simulink model "KF_3_gdl_AHRS_Dataset2"  (R2020b)
settings: Solver=FixedStepAuto  StartTime=0.0  StopTime=1000  FixedStep=1/200  RelTol=1e-3
values from neighbouring files (symbols this model uses):
  BARO_cov = single(1.7)/2    [init_1gdl.m]    (also in init_3_gdl_AHRS_fb.m = single(1.7)/5; init_3gdl.m; init_dati_veri.m = single(1.7)/5)
  BARO_cov_old = single(1.7)/2    [init_1gdl.m]    (also in init_3_gdl_AHRS_fb.m; init_3gdl.m; init_dati_veri.m)
  bj_x = 0.4    [init_3_gdl_AHRS_fb.m]
  bj_y = 0.9    [init_3_gdl_AHRS_fb.m]
  bj_z = 0.5    [init_3_gdl_AHRS_fb.m]
  bjy = bj_y - 0.1    (= 0.8)    [init_3_gdl_AHRS_fb.m]
  filter_pos = tf(1,[1 1])    [init_1gdl.m]    (also in init_3_gdl_AHRS_fb.m; init_3gdl.m; init_dati_veri.m)
  filter_pos_Z = tf(1,[0.5 1])    [init_3_gdl_AHRS_fb.m]    (also in init_3gdl.m; init_dati_veri.m)
  g_ned = [0; 0; -9.81]    [init_3_gdl_AHRS_fb.m]    (also in init_dati_veri.m)
  GPS_cov = single([1*2, 1])/2    [init_1gdl.m]    (also in init_3_gdl_AHRS_fb.m = single([0.1*50, 0.1*50, 200*5, 200*5, 0.36])/2; init_3gdl.m = single([1*2, 1*2, 1, 1, 0.36])/2; init_dati_veri.m = single([0.1, 0.1, 200*5, 200*5, 0.36])/2)
  GPS_cov_old = single([0.1, 0.1, 200, 200, 0.36])/2    [init_1gdl.m]    (also in init_3_gdl_AHRS_fb.m = single([0.1, 0.1, 200, 200, 0.36]/2); init_3gdl.m; init_dati_veri.m = single([0.1, 0.1, 200, 200, 0.36]/2))
  IMU_cov = single(15*0.07)/2    [init_1gdl.m]    (also in init_3_gdl_AHRS_fb.m = single([15*[0.07*50, 0.07*50] 15*50*0.09])/2; init_3gdl.m = single([15*[0.07, 0.07] 10*0.09])/2; init_dati_veri.m = single([15*[0.07*5, 0.07*5] 15*50*0.09])/2)
  IMU_cov_old = single([15*[0.07, 0.07] 10*0.09])/2    [init_1gdl.m]    (also in init_3_gdl_AHRS_fb.m = single([15*[0.07, 0.07] 10*0.09]/2); init_3gdl.m; init_dati_veri.m = single([15*[0.07, 0.07] 10*0.09]/2))
  Q = single(diag([1e-2, 1e-6, 1e-4, 1e-12]))*2    [init_1gdl.m]    (also in init_3_gdl_AHRS_fb.m = single(diag([px,vx,ax,py,vy,ay,pz,vz,az,bx,by,bz]))*2; init_3gdl.m = single(diag([px,vx,ax,py,vy,ay,pz,vz,az,bx,by,bz]))*2; init_dati_veri.m = single(diag([px,vx,ax,py,vy,ay,pz,vz,az,bx,by,bz]))*2)
  Q_old = single(diag([1e-8, 1e-1, 1e-2, 1e-8, 1e-1, 1e-2, 1e-5, 1e-4, 0.010]))*2    [init_1gdl.m]    (also in init_3_gdl_AHRS_fb.m; init_3gdl.m; init_dati_veri.m)
  ST = 1/200    (= 0.005)    [init_1gdl.m]    (also in init_3_gdl_AHRS_fb.m; init_3gdl.m; init_dati_veri.m)
  T_50 = 1/50    (= 0.02)    [init_1gdl.m]    (also in init_3_gdl_AHRS_fb.m; init_3gdl.m; init_dati_veri.m)
  var_giroscopio = [(deg2rad(0.16))^2;(deg2rad(0.16))^2;(deg2rad(0.16))^2]    [init_3_gdl_AHRS_fb.m]    (also in init_dati_veri.m)
  var_p_x = 2    [init_3_gdl_AHRS_fb.m]    (also in init_3gdl.m = 1; init_dati_veri.m)
  var_p_y = 2    [init_3_gdl_AHRS_fb.m]    (also in init_3gdl.m = 1; init_dati_veri.m)
  var_p_z = 0.30    (= 0.3)    [init_3_gdl_AHRS_fb.m]    (also in init_3gdl.m = 0.15; init_dati_veri.m)
  var_v_x = 0.60    (= 0.6)    [init_3_gdl_AHRS_fb.m]    (also in init_3gdl.m = 0.3; init_dati_veri.m)
  var_v_y = 0.32    [init_3_gdl_AHRS_fb.m]    (also in init_3gdl.m = 0.16; init_dati_veri.m)
  var_v_z = 0.60    (= 0.6)    [init_3_gdl_AHRS_fb.m]    (also in init_3gdl.m = 0.3; init_dati_veri.m)
undefined symbols (not defined in the file or in its folder): DiscIntNeverNeededParam
libraries: simulink x33, cstblocks x9
(part 2 of 4)

== system KF_3_gdl_AHRS_Dataset2/MPU AHRS1/debias MPU ==
  acc : Inport
  gyros : Inport  Port=2
  "Acceleration Detrend " : Subsystem  mask{ST2=ST}
      mask prompts: ST2 "Sample Time"
  Add : Sum  Inputs=+-
  Data Type Conversion mx1 : DataTypeConversion  OutDataTypeStr=boolean  RndMeth=Round  SaturateOnIntegerOverflow=on
  Data Type Conversion mx8 : DataTypeConversion  OutDataTypeStr=single  RndMeth=Round  SaturateOnIntegerOverflow=on
  Gyros Detrend : Subsystem  mask{ST2=ST}
      mask prompts: ST2 "Sample Time"
  Step : Step  SampleTime=ST
  Step1 : Step  Time=11  SampleTime=ST
  acc_out : Outport
  gyro_out : Outport  Port=2
  detrending_ok : Outport  Port=3
  wires:
  Step/1 -> Add/1
  Step1/1 -> Add/2, Data Type Conversion mx1/1
  Add/1 -> Data Type Conversion mx8/1
  acc/1 -> "Acceleration Detrend "/1(In)
  gyros/1 -> Gyros Detrend/1(In)
  "Acceleration Detrend "/1(Out) -> acc_out/1
  Gyros Detrend/1(Out) -> gyro_out/1
  Data Type Conversion mx1/1 -> detrending_ok/1
  Data Type Conversion mx8/1 -> Gyros Detrend/2(Detrending), "Acceleration Detrend "/2(Detrending)

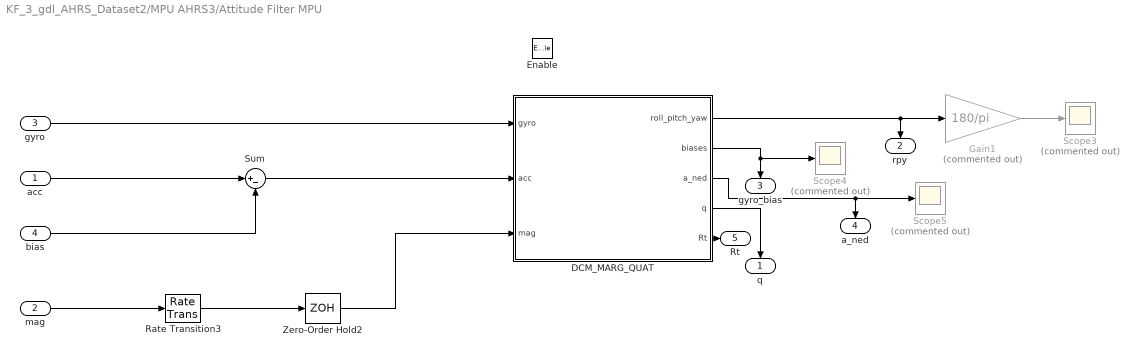
== system KF_3_gdl_AHRS_Dataset2/MPU AHRS3/Attitude Filter MPU ==
  acc : Inport
  mag : Inport  Port=2
  gyro : Inport  Port=3
  bias : Inport  Port=4
  Enable : EnablePort  StatesWhenEnabling=reset
  DCM_MARG_QUAT : Subsystem  mask{Kp=0.15*0, Ki=0, tau=40, T=T}
      mask prompts: Kp "Proportional Gain"; Ki "Integral Gain"; tau "Biases Time Constant"; T "Sample Time"
  Gain1 : Gain  Commented=on  Gain=180/pi
  Rate Transition3 : RateTransition  Deterministic=off
  Scope3 : Scope  Commented=on
  Scope4 : Scope  Commented=on
  Scope5 : Scope  Commented=on
  Sum : Sum  Inputs=|+-
  Zero-Order Hold2 : ZeroOrderHold  SampleTime=T
  q : Outport  PortDimensions=4  InitialOutput=[1 0 0 0]'
  rpy : Outport  Port=2  PortDimensions=3  InitialOutput=[0 0 0]'
  gyro_bias : Outport  Port=3  PortDimensions=3  InitialOutput=[0 0 0]'
  a_ned : Outport  Port=4  InitialOutput=[0 0 0]'
  Rt : Outport  Port=5
  wires:
  Rate Transition3/1 -> Zero-Order Hold2/1
  Zero-Order Hold2/1 -> DCM_MARG_QUAT/3(mag)
  DCM_MARG_QUAT/4(q) -> q/1
  bias/1 -> Sum/2
  Sum/1 -> DCM_MARG_QUAT/2(acc)
  acc/1 -> Sum/1
  DCM_MARG_QUAT/3(a_ned) -> a_ned/1, Scope5/1
  DCM_MARG_QUAT/1(roll_pitch_yaw) -> rpy/1, Gain1/1
  mag/1 -> Rate Transition3/1
  gyro/1 -> DCM_MARG_QUAT/1(gyro)
  DCM_MARG_QUAT/2(biases) -> gyro_bias/1, Scope4/1
  Gain1/1 -> Scope3/1
  DCM_MARG_QUAT/5(Rt) -> Rt/1

== system KF_3_gdl_AHRS_Dataset2/MPU AHRS3/debias MPU ==
  acc : Inport
  gyros : Inport  Port=2
  "Acceleration Detrend " : Subsystem  mask{ST2=ST}
      mask prompts: ST2 "Sample Time"
  Add : Sum  Inputs=+-
  Data Type Conversion mx1 : DataTypeConversion  OutDataTypeStr=boolean  RndMeth=Round  SaturateOnIntegerOverflow=on
  Data Type Conversion mx8 : DataTypeConversion  OutDataTypeStr=single  RndMeth=Round  SaturateOnIntegerOverflow=on
  Gyros Detrend : Subsystem  mask{ST2=ST}
      mask prompts: ST2 "Sample Time"
  Step : Step  SampleTime=ST
  Step1 : Step  Time=11  SampleTime=ST
  acc_out : Outport
  gyro_out : Outport  Port=2
  detrending_ok : Outport  Port=3
  wires:
  Step/1 -> Add/1
  Step1/1 -> Add/2, Data Type Conversion mx1/1
  Add/1 -> Data Type Conversion mx8/1
  acc/1 -> "Acceleration Detrend "/1(In)
  gyros/1 -> Gyros Detrend/1(In)
  "Acceleration Detrend "/1(Out) -> acc_out/1
  Gyros Detrend/1(Out) -> gyro_out/1
  Data Type Conversion mx8/1 -> "Acceleration Detrend "/2(Detrending), Gyros Detrend/2(Detrending)
  Data Type Conversion mx1/1 -> detrending_ok/1

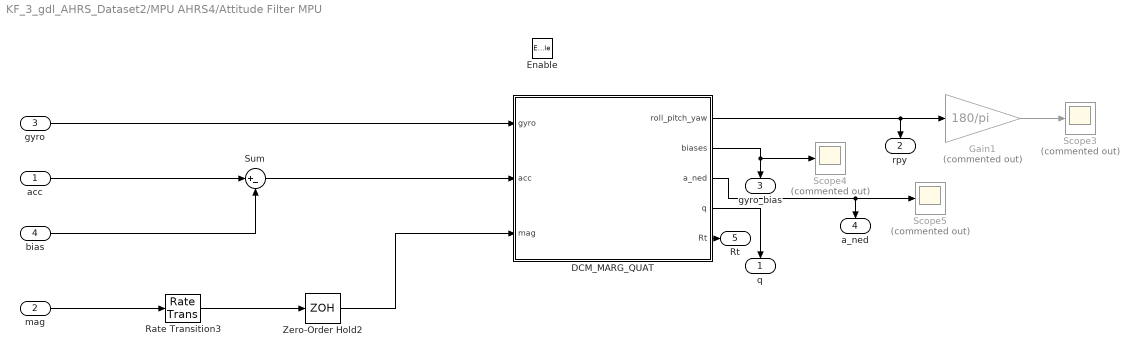
== system KF_3_gdl_AHRS_Dataset2/MPU AHRS4/Attitude Filter MPU ==
  acc : Inport
  mag : Inport  Port=2
  gyro : Inport  Port=3
  bias : Inport  Port=4
  Enable : EnablePort  StatesWhenEnabling=reset
  DCM_MARG_QUAT : Subsystem  mask{Kp=0.15, Ki=0, tau=40, T=T}
      mask prompts: Kp "Proportional Gain"; Ki "Integral Gain"; tau "Biases Time Constant"; T "Sample Time"
  Gain1 : Gain  Commented=on  Gain=180/pi
  Rate Transition3 : RateTransition  Deterministic=off
  Scope3 : Scope  Commented=on
  Scope4 : Scope  Commented=on
  Scope5 : Scope  Commented=on
  Sum : Sum  Inputs=|+-
  Zero-Order Hold2 : ZeroOrderHold  SampleTime=T
  q : Outport  PortDimensions=4  InitialOutput=[1 0 0 0]'
  rpy : Outport  Port=2  PortDimensions=3  InitialOutput=[0 0 0]'
  gyro_bias : Outport  Port=3  PortDimensions=3  InitialOutput=[0 0 0]'
  a_ned : Outport  Port=4  InitialOutput=[0 0 0]'
  Rt : Outport  Port=5
  wires:
  Rate Transition3/1 -> Zero-Order Hold2/1
  Zero-Order Hold2/1 -> DCM_MARG_QUAT/3(mag)
  DCM_MARG_QUAT/4(q) -> q/1
  bias/1 -> Sum/2
  Sum/1 -> DCM_MARG_QUAT/2(acc)
  acc/1 -> Sum/1
  DCM_MARG_QUAT/3(a_ned) -> a_ned/1, Scope5/1
  DCM_MARG_QUAT/1(roll_pitch_yaw) -> rpy/1, Gain1/1
  mag/1 -> Rate Transition3/1
  gyro/1 -> DCM_MARG_QUAT/1(gyro)
  DCM_MARG_QUAT/2(biases) -> gyro_bias/1, Scope4/1
  Gain1/1 -> Scope3/1
  DCM_MARG_QUAT/5(Rt) -> Rt/1

== system KF_3_gdl_AHRS_Dataset2/MPU AHRS4/debias MPU ==
  acc : Inport
  gyros : Inport  Port=2
  "Acceleration Detrend " : Subsystem  mask{ST2=ST}
      mask prompts: ST2 "Sample Time"
  Add : Sum  Inputs=+-
  Data Type Conversion mx1 : DataTypeConversion  OutDataTypeStr=boolean  RndMeth=Round  SaturateOnIntegerOverflow=on
  Data Type Conversion mx8 : DataTypeConversion  OutDataTypeStr=single  RndMeth=Round  SaturateOnIntegerOverflow=on
  Gyros Detrend : Subsystem  mask{ST2=ST}
      mask prompts: ST2 "Sample Time"
  Step : Step  SampleTime=ST
  Step1 : Step  Time=11  SampleTime=ST
  acc_out : Outport
  gyro_out : Outport  Port=2
  detrending_ok : Outport  Port=3
  wires:
  Step/1 -> Add/1
  Step1/1 -> Add/2, Data Type Conversion mx1/1
  Add/1 -> Data Type Conversion mx8/1
  acc/1 -> "Acceleration Detrend "/1(In)
  gyros/1 -> Gyros Detrend/1(In)
  "Acceleration Detrend "/1(Out) -> acc_out/1
  Gyros Detrend/1(Out) -> gyro_out/1
  Data Type Conversion mx1/1 -> detrending_ok/1
  Data Type Conversion mx8/1 -> Gyros Detrend/2(Detrending), "Acceleration Detrend "/2(Detrending)

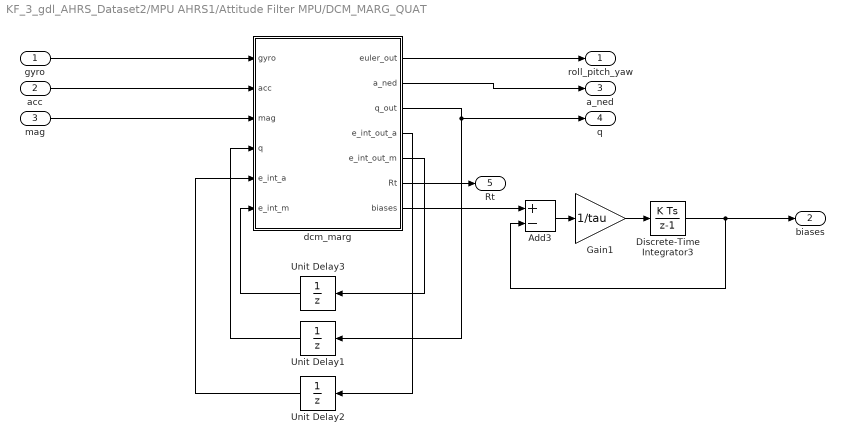
== system KF_3_gdl_AHRS_Dataset2/MPU AHRS1/Attitude Filter MPU/DCM_MARG_QUAT ==
  gyro : Inport
  acc : Inport  Port=2
  mag : Inport  Port=3
  Add3 : Sum  Inputs=+-
  Discrete-Time Integrator3 : DiscreteIntegrator  SampleTime=T  ICPrevOutput=DiscIntNeverNeededParam  ICPrevScaledInput=DiscIntNeverNeededParam
  Gain1 : Gain  Gain=1/tau  ParamDataTypeStr=single  OutDataTypeStr=single
  Unit Delay1 : UnitDelay  InitialCondition=[1;0;0;0]  SampleTime=T  HasFrameUpgradeWarning=on
  Unit Delay2 : UnitDelay  SampleTime=T  HasFrameUpgradeWarning=on
  Unit Delay3 : UnitDelay  SampleTime=T  HasFrameUpgradeWarning=on
  dcm_marg : MATLAB Function  TreatAsAtomicUnit=on
  roll_pitch_yaw : Outport
  biases : Outport  Port=2
  a_ned : Outport  Port=3
  q : Outport  Port=4
  Rt : Outport  Port=5
  wires:
  Unit Delay3/1 -> dcm_marg/6(e_int_m)
  dcm_marg/5(e_int_out_m) -> Unit Delay3/1
  dcm_marg/2(a_ned) -> a_ned/1
  Discrete-Time Integrator3/1 -> biases/1, Add3/2
  Gain1/1 -> Discrete-Time Integrator3/1
  Add3/1 -> Gain1/1
  dcm_marg/1(euler_out) -> roll_pitch_yaw/1
  gyro/1 -> dcm_marg/1(gyro)
  acc/1 -> dcm_marg/2(acc)
  mag/1 -> dcm_marg/3(mag)
  dcm_marg/3(q_out) -> q/1, Unit Delay1/1
  Unit Delay1/1 -> dcm_marg/4(q)
  dcm_marg/4(e_int_out_a) -> Unit Delay2/1
  Unit Delay2/1 -> dcm_marg/5(e_int_a)
  dcm_marg/7(biases) -> Add3/1
  dcm_marg/6(Rt) -> Rt/1

== system KF_3_gdl_AHRS_Dataset2/MPU AHRS1/debias MPU/Acceleration Detrend  ==
  In : Inport
  Detrending : Inport  Port=2
  Demux : Demux  Outputs=3
      settings: DisplayOption=none
  Detrend : Subsystem  mask{ST=ST2}
      mask prompts: ST "Sample Time"
  Detrend1 : Subsystem  mask{ST=ST2}
      mask prompts: ST "Sample Time"
  Detrend3 : Subsystem  mask{ST=ST2}
      mask prompts: ST "Sample Time"
  Mux : Mux  Inputs=3
  Out : Outport
  wires:
  Detrending/1 -> Detrend3/2(Detrending), Detrend1/2(Detrending), Detrend/2(Detrending)
  Demux/3 -> Detrend3/1(Input)
  In/1 -> Demux/1
  Demux/2 -> Detrend1/1(Input)
  Demux/1 -> Detrend/1(Input)
  Mux/1 -> Out/1
  Detrend3/1(Detrended Output) -> Mux/3
  Detrend1/1(Detrended Output) -> Mux/2
  Detrend/1(Detrended Output) -> Mux/1

== system KF_3_gdl_AHRS_Dataset2/MPU AHRS1/debias MPU/Gyros Detrend ==
  In : Inport
  Detrending : Inport  Port=2
  Demux : Demux  Outputs=3
      settings: DisplayOption=none
  Detrend : Subsystem  mask{ST=ST2}
      mask prompts: ST "Sample Time"
  Detrend2 : Subsystem  mask{ST=ST2}
      mask prompts: ST "Sample Time"
  Detrend3 : Subsystem  mask{ST=ST2}
      mask prompts: ST "Sample Time"
  Mux : Mux  Inputs=3
  Out : Outport
  wires:
  Detrend/1(Detrended Output) -> Mux/1
  Detrend3/1(Detrended Output) -> Mux/2
  Detrend2/1(Detrended Output) -> Mux/3
  Mux/1 -> Out/1
  Demux/1 -> Detrend/1(Input)
  Demux/2 -> Detrend3/1(Input)
  In/1 -> Demux/1
  Demux/3 -> Detrend2/1(Input)
  Detrending/1 -> Detrend2/2(Detrending), Detrend3/2(Detrending), Detrend/2(Detrending)

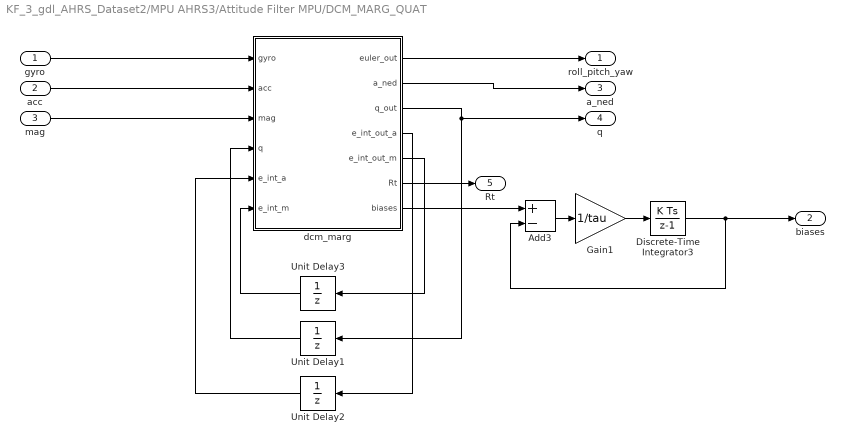
== system KF_3_gdl_AHRS_Dataset2/MPU AHRS3/Attitude Filter MPU/DCM_MARG_QUAT ==
  gyro : Inport
  acc : Inport  Port=2
  mag : Inport  Port=3
  Add3 : Sum  Inputs=+-
  Discrete-Time Integrator3 : DiscreteIntegrator  SampleTime=T  ICPrevOutput=DiscIntNeverNeededParam  ICPrevScaledInput=DiscIntNeverNeededParam
  Gain1 : Gain  Gain=1/tau  ParamDataTypeStr=single  OutDataTypeStr=single
  Unit Delay1 : UnitDelay  InitialCondition=[1;0;0;0]  SampleTime=T  HasFrameUpgradeWarning=on
  Unit Delay2 : UnitDelay  SampleTime=T  HasFrameUpgradeWarning=on
  Unit Delay3 : UnitDelay  SampleTime=T  HasFrameUpgradeWarning=on
  dcm_marg : MATLAB Function  TreatAsAtomicUnit=on
  roll_pitch_yaw : Outport
  biases : Outport  Port=2
  a_ned : Outport  Port=3
  q : Outport  Port=4
  Rt : Outport  Port=5
  wires:
  Unit Delay3/1 -> dcm_marg/6(e_int_m)
  dcm_marg/5(e_int_out_m) -> Unit Delay3/1
  dcm_marg/2(a_ned) -> a_ned/1
  Discrete-Time Integrator3/1 -> biases/1, Add3/2
  Gain1/1 -> Discrete-Time Integrator3/1
  Add3/1 -> Gain1/1
  dcm_marg/1(euler_out) -> roll_pitch_yaw/1
  gyro/1 -> dcm_marg/1(gyro)
  acc/1 -> dcm_marg/2(acc)
  mag/1 -> dcm_marg/3(mag)
  dcm_marg/3(q_out) -> q/1, Unit Delay1/1
  Unit Delay1/1 -> dcm_marg/4(q)
  dcm_marg/4(e_int_out_a) -> Unit Delay2/1
  Unit Delay2/1 -> dcm_marg/5(e_int_a)
  dcm_marg/7(biases) -> Add3/1
  dcm_marg/6(Rt) -> Rt/1

== system KF_3_gdl_AHRS_Dataset2/MPU AHRS3/debias MPU/Acceleration Detrend  ==
  In : Inport
  Detrending : Inport  Port=2
  Demux : Demux  Outputs=3
      settings: DisplayOption=none
  Detrend : Subsystem  mask{ST=ST2}
      mask prompts: ST "Sample Time"
  Detrend1 : Subsystem  mask{ST=ST2}
      mask prompts: ST "Sample Time"
  Detrend3 : Subsystem  mask{ST=ST2}
      mask prompts: ST "Sample Time"
  Mux : Mux  Inputs=3
  Out : Outport
  wires:
  Detrending/1 -> Detrend3/2(Detrending), Detrend1/2(Detrending), Detrend/2(Detrending)
  Demux/3 -> Detrend3/1(Input)
  In/1 -> Demux/1
  Demux/2 -> Detrend1/1(Input)
  Demux/1 -> Detrend/1(Input)
  Mux/1 -> Out/1
  Detrend3/1(Detrended Output) -> Mux/3
  Detrend1/1(Detrended Output) -> Mux/2
  Detrend/1(Detrended Output) -> Mux/1

== system KF_3_gdl_AHRS_Dataset2/MPU AHRS3/debias MPU/Gyros Detrend ==
  In : Inport
  Detrending : Inport  Port=2
  Demux : Demux  Outputs=3
      settings: DisplayOption=none
  Detrend : Subsystem  mask{ST=ST2}
      mask prompts: ST "Sample Time"
  Detrend2 : Subsystem  mask{ST=ST2}
      mask prompts: ST "Sample Time"
  Detrend3 : Subsystem  mask{ST=ST2}
      mask prompts: ST "Sample Time"
  Mux : Mux  Inputs=3
  Out : Outport
  wires:
  Detrend/1(Detrended Output) -> Mux/1
  Detrend3/1(Detrended Output) -> Mux/2
  Detrend2/1(Detrended Output) -> Mux/3
  Mux/1 -> Out/1
  Demux/1 -> Detrend/1(Input)
  Demux/2 -> Detrend3/1(Input)
  In/1 -> Demux/1
  Demux/3 -> Detrend2/1(Input)
  Detrending/1 -> Detrend2/2(Detrending), Detrend3/2(Detrending), Detrend/2(Detrending)

== system KF_3_gdl_AHRS_Dataset2/MPU AHRS4/Attitude Filter MPU/DCM_MARG_QUAT ==
  gyro : Inport
  acc : Inport  Port=2
  mag : Inport  Port=3
  Add3 : Sum  Inputs=+-
  Discrete-Time Integrator3 : DiscreteIntegrator  SampleTime=T  ICPrevOutput=DiscIntNeverNeededParam  ICPrevScaledInput=DiscIntNeverNeededParam
  Gain1 : Gain  Gain=1/tau  ParamDataTypeStr=single  OutDataTypeStr=single
  Unit Delay1 : UnitDelay  InitialCondition=[1;0;0;0]  SampleTime=T  HasFrameUpgradeWarning=on
  Unit Delay2 : UnitDelay  SampleTime=T  HasFrameUpgradeWarning=on
  Unit Delay3 : UnitDelay  SampleTime=T  HasFrameUpgradeWarning=on
  dcm_marg : MATLAB Function  TreatAsAtomicUnit=on
  roll_pitch_yaw : Outport
  biases : Outport  Port=2
  a_ned : Outport  Port=3
  q : Outport  Port=4
  Rt : Outport  Port=5
  wires:
  Unit Delay3/1 -> dcm_marg/6(e_int_m)
  dcm_marg/5(e_int_out_m) -> Unit Delay3/1
  dcm_marg/2(a_ned) -> a_ned/1
  Discrete-Time Integrator3/1 -> biases/1, Add3/2
  Gain1/1 -> Discrete-Time Integrator3/1
  Add3/1 -> Gain1/1
  dcm_marg/1(euler_out) -> roll_pitch_yaw/1
  gyro/1 -> dcm_marg/1(gyro)
  acc/1 -> dcm_marg/2(acc)
  mag/1 -> dcm_marg/3(mag)
  dcm_marg/3(q_out) -> q/1, Unit Delay1/1
  Unit Delay1/1 -> dcm_marg/4(q)
  dcm_marg/4(e_int_out_a) -> Unit Delay2/1
  Unit Delay2/1 -> dcm_marg/5(e_int_a)
  dcm_marg/7(biases) -> Add3/1
  dcm_marg/6(Rt) -> Rt/1

== system KF_3_gdl_AHRS_Dataset2/MPU AHRS4/debias MPU/Acceleration Detrend  ==
  In : Inport
  Detrending : Inport  Port=2
  Demux : Demux  Outputs=3
      settings: DisplayOption=none
  Detrend : Subsystem  mask{ST=ST2}
      mask prompts: ST "Sample Time"
  Detrend1 : Subsystem  mask{ST=ST2}
      mask prompts: ST "Sample Time"
  Detrend3 : Subsystem  mask{ST=ST2}
      mask prompts: ST "Sample Time"
  Mux : Mux  Inputs=3
  Out : Outport
  wires:
  Detrending/1 -> Detrend3/2(Detrending), Detrend1/2(Detrending), Detrend/2(Detrending)
  Demux/3 -> Detrend3/1(Input)
  In/1 -> Demux/1
  Demux/2 -> Detrend1/1(Input)
  Demux/1 -> Detrend/1(Input)
  Mux/1 -> Out/1
  Detrend3/1(Detrended Output) -> Mux/3
  Detrend1/1(Detrended Output) -> Mux/2
  Detrend/1(Detrended Output) -> Mux/1

== system KF_3_gdl_AHRS_Dataset2/MPU AHRS4/debias MPU/Gyros Detrend ==
  In : Inport
  Detrending : Inport  Port=2
  Demux : Demux  Outputs=3
      settings: DisplayOption=none
  Detrend : Subsystem  mask{ST=ST2}
      mask prompts: ST "Sample Time"
  Detrend2 : Subsystem  mask{ST=ST2}
      mask prompts: ST "Sample Time"
  Detrend3 : Subsystem  mask{ST=ST2}
      mask prompts: ST "Sample Time"
  Mux : Mux  Inputs=3
  Out : Outport
  wires:
  Detrend/1(Detrended Output) -> Mux/1
  Detrend3/1(Detrended Output) -> Mux/2
  Detrend2/1(Detrended Output) -> Mux/3
  Mux/1 -> Out/1
  Demux/1 -> Detrend/1(Input)
  Demux/2 -> Detrend3/1(Input)
  In/1 -> Demux/1
  Demux/3 -> Detrend2/1(Input)
  Detrending/1 -> Detrend2/2(Detrending), Detrend3/2(Detrending), Detrend/2(Detrending)

== system KF_3_gdl_AHRS_Dataset2/MPU AHRS1/debias MPU/Acceleration Detrend /Detrend ==
  Input : Inport
  Detrending : Inport  Port=2
  Compare To Constant : simulink/Logic and Bit Operations/Compare To Constant  relop=>=  const=0.5  OutDataTypeStr=boolean
  Constant1 : Constant  Value=0  OutDataTypeStr=single
  Subsystem : Subsystem  TreatAsAtomicUnit=on
  Sum1 : Sum  Inputs=|+-  InputSameDT=on  SaturateOnIntegerOverflow=on  OutDataTypeStr=Inherit: Same as first input
  Switch2 : Switch  Threshold=0.5  SaturateOnIntegerOverflow=on  InputSameDT=on
  Detrended Output : Outport
  wires:
  Switch2/1 -> Detrended Output/1
  Detrending/1 -> Switch2/2, Compare To Constant/1
  Subsystem/1(Out2) -> Sum1/2
  Constant1/1 -> Switch2/1
  Input/1 -> Sum1/1, Subsystem/1(In1)
  Sum1/1 -> Switch2/3
  Compare To Constant/1 -> Subsystem/Enable

== system KF_3_gdl_AHRS_Dataset2/MPU AHRS1/debias MPU/Acceleration Detrend /Detrend1 ==
  Input : Inport
  Detrending : Inport  Port=2
  Compare To Constant : simulink/Logic and Bit Operations/Compare To Constant  relop=>=  const=0.5  OutDataTypeStr=boolean
  Constant1 : Constant  Value=0  OutDataTypeStr=single
  Subsystem : Subsystem  TreatAsAtomicUnit=on
  Sum1 : Sum  Inputs=|+-  InputSameDT=on  SaturateOnIntegerOverflow=on  OutDataTypeStr=Inherit: Same as first input
  Switch2 : Switch  Threshold=0.5  SaturateOnIntegerOverflow=on  InputSameDT=on
  Detrended Output : Outport
  wires:
  Compare To Constant/1 -> Subsystem/Enable
  Sum1/1 -> Switch2/3
  Input/1 -> Subsystem/1(In1), Sum1/1
  Constant1/1 -> Switch2/1
  Subsystem/1(Out2) -> Sum1/2
  Detrending/1 -> Compare To Constant/1, Switch2/2
  Switch2/1 -> Detrended Output/1

== system KF_3_gdl_AHRS_Dataset2/MPU AHRS1/debias MPU/Acceleration Detrend /Detrend3 ==
  Input : Inport
  Detrending : Inport  Port=2
  Compare To Constant : simulink/Logic and Bit Operations/Compare To Constant  relop=>=  const=0.5  OutDataTypeStr=boolean
  Constant1 : Constant  Value=0  OutDataTypeStr=single
  Constant2 : Constant  Value=9.81  OutDataTypeStr=single
  Subsystem : Subsystem  TreatAsAtomicUnit=on
  Sum1 : Sum  Inputs=|+--  InputSameDT=on  SaturateOnIntegerOverflow=on  OutDataTypeStr=Inherit: Same as first input
  Switch2 : Switch  Threshold=0.5  SaturateOnIntegerOverflow=on  InputSameDT=on
  Detrended Output : Outport
  wires:
  Switch2/1 -> Detrended Output/1
  Detrending/1 -> Switch2/2, Compare To Constant/1
  Subsystem/1(Out2) -> Sum1/2
  Constant1/1 -> Switch2/1
  Input/1 -> Sum1/1, Subsystem/1(In1)
  Sum1/1 -> Switch2/3
  Compare To Constant/1 -> Subsystem/Enable
  Constant2/1 -> Sum1/3

== system KF_3_gdl_AHRS_Dataset2/MPU AHRS1/debias MPU/Gyros Detrend/Detrend ==
  Input : Inport
  Detrending : Inport  Port=2
  Compare To Constant : simulink/Logic and Bit Operations/Compare To Constant  relop=>=  const=0.5  OutDataTypeStr=boolean
  Constant1 : Constant  Value=0  OutDataTypeStr=single
  Subsystem : Subsystem  TreatAsAtomicUnit=on
  Sum1 : Sum  Inputs=|+-  InputSameDT=on  SaturateOnIntegerOverflow=on  OutDataTypeStr=Inherit: Same as first input
  Switch2 : Switch  Threshold=0.5  SaturateOnIntegerOverflow=on  InputSameDT=on
  Detrended Output : Outport
  wires:
  Switch2/1 -> Detrended Output/1
  Detrending/1 -> Switch2/2, Compare To Constant/1
  Subsystem/1(Out2) -> Sum1/2
  Constant1/1 -> Switch2/1
  Input/1 -> Sum1/1, Subsystem/1(In1)
  Sum1/1 -> Switch2/3
  Compare To Constant/1 -> Subsystem/Enable

== system KF_3_gdl_AHRS_Dataset2/MPU AHRS1/debias MPU/Gyros Detrend/Detrend2 ==
  Input : Inport
  Detrending : Inport  Port=2
  Compare To Constant : simulink/Logic and Bit Operations/Compare To Constant  relop=>=  const=0.5  OutDataTypeStr=boolean
  Constant1 : Constant  Value=0  OutDataTypeStr=single
  Subsystem : Subsystem  TreatAsAtomicUnit=on
  Sum1 : Sum  Inputs=|+-  InputSameDT=on  SaturateOnIntegerOverflow=on  OutDataTypeStr=Inherit: Same as first input
  Switch2 : Switch  Threshold=0.5  SaturateOnIntegerOverflow=on  InputSameDT=on
  Detrended Output : Outport
  wires:
  Switch2/1 -> Detrended Output/1
  Detrending/1 -> Switch2/2, Compare To Constant/1
  Subsystem/1(Out2) -> Sum1/2
  Constant1/1 -> Switch2/1
  Input/1 -> Sum1/1, Subsystem/1(In1)
  Sum1/1 -> Switch2/3
  Compare To Constant/1 -> Subsystem/Enable

== system KF_3_gdl_AHRS_Dataset2/MPU AHRS1/debias MPU/Gyros Detrend/Detrend3 ==
  Input : Inport
  Detrending : Inport  Port=2
  Compare To Constant : simulink/Logic and Bit Operations/Compare To Constant  relop=>=  const=0.5  OutDataTypeStr=boolean
  Constant1 : Constant  Value=0  OutDataTypeStr=single
  Subsystem : Subsystem  TreatAsAtomicUnit=on
  Sum1 : Sum  Inputs=|+-  InputSameDT=on  SaturateOnIntegerOverflow=on  OutDataTypeStr=Inherit: Same as first input
  Switch2 : Switch  Threshold=0.5  SaturateOnIntegerOverflow=on  InputSameDT=on
  Detrended Output : Outport
  wires:
  Compare To Constant/1 -> Subsystem/Enable
  Sum1/1 -> Switch2/3
  Input/1 -> Subsystem/1(In1), Sum1/1
  Constant1/1 -> Switch2/1
  Subsystem/1(Out2) -> Sum1/2
  Detrending/1 -> Compare To Constant/1, Switch2/2
  Switch2/1 -> Detrended Output/1

== system KF_3_gdl_AHRS_Dataset2/MPU AHRS3/debias MPU/Acceleration Detrend /Detrend ==
  Input : Inport
  Detrending : Inport  Port=2
  Compare To Constant : simulink/Logic and Bit Operations/Compare To Constant  relop=>=  const=0.5  OutDataTypeStr=boolean
  Constant1 : Constant  Value=0  OutDataTypeStr=single
  Subsystem : Subsystem  TreatAsAtomicUnit=on
  Sum1 : Sum  Inputs=|+-  InputSameDT=on  SaturateOnIntegerOverflow=on  OutDataTypeStr=Inherit: Same as first input
  Switch2 : Switch  Threshold=0.5  SaturateOnIntegerOverflow=on  InputSameDT=on
  Detrended Output : Outport
  wires:
  Switch2/1 -> Detrended Output/1
  Detrending/1 -> Switch2/2, Compare To Constant/1
  Subsystem/1(Out2) -> Sum1/2
  Constant1/1 -> Switch2/1
  Input/1 -> Sum1/1, Subsystem/1(In1)
  Sum1/1 -> Switch2/3
  Compare To Constant/1 -> Subsystem/Enable

== system KF_3_gdl_AHRS_Dataset2/MPU AHRS3/debias MPU/Acceleration Detrend /Detrend1 ==
  Input : Inport
  Detrending : Inport  Port=2
  Compare To Constant : simulink/Logic and Bit Operations/Compare To Constant  relop=>=  const=0.5  OutDataTypeStr=boolean
  Constant1 : Constant  Value=0  OutDataTypeStr=single
  Subsystem : Subsystem  TreatAsAtomicUnit=on
  Sum1 : Sum  Inputs=|+-  InputSameDT=on  SaturateOnIntegerOverflow=on  OutDataTypeStr=Inherit: Same as first input
  Switch2 : Switch  Threshold=0.5  SaturateOnIntegerOverflow=on  InputSameDT=on
  Detrended Output : Outport
  wires:
  Compare To Constant/1 -> Subsystem/Enable
  Sum1/1 -> Switch2/3
  Input/1 -> Subsystem/1(In1), Sum1/1
  Constant1/1 -> Switch2/1
  Subsystem/1(Out2) -> Sum1/2
  Detrending/1 -> Compare To Constant/1, Switch2/2
  Switch2/1 -> Detrended Output/1

== system KF_3_gdl_AHRS_Dataset2/MPU AHRS3/debias MPU/Acceleration Detrend /Detrend3 ==
  Input : Inport
  Detrending : Inport  Port=2
  Compare To Constant : simulink/Logic and Bit Operations/Compare To Constant  relop=>=  const=0.5  OutDataTypeStr=boolean
  Constant1 : Constant  Value=0  OutDataTypeStr=single
  Constant2 : Constant  Value=9.81  OutDataTypeStr=single
  Subsystem : Subsystem  TreatAsAtomicUnit=on
  Sum1 : Sum  Inputs=|+--  InputSameDT=on  SaturateOnIntegerOverflow=on  OutDataTypeStr=Inherit: Same as first input
  Switch2 : Switch  Threshold=0.5  SaturateOnIntegerOverflow=on  InputSameDT=on
  Detrended Output : Outport
  wires:
  Switch2/1 -> Detrended Output/1
  Detrending/1 -> Switch2/2, Compare To Constant/1
  Subsystem/1(Out2) -> Sum1/2
  Constant1/1 -> Switch2/1
  Input/1 -> Sum1/1, Subsystem/1(In1)
  Sum1/1 -> Switch2/3
  Compare To Constant/1 -> Subsystem/Enable
  Constant2/1 -> Sum1/3

== system KF_3_gdl_AHRS_Dataset2/MPU AHRS3/debias MPU/Gyros Detrend/Detrend ==
  Input : Inport
  Detrending : Inport  Port=2
  Compare To Constant : simulink/Logic and Bit Operations/Compare To Constant  relop=>=  const=0.5  OutDataTypeStr=boolean
  Constant1 : Constant  Value=0  OutDataTypeStr=single
  Subsystem : Subsystem  TreatAsAtomicUnit=on
  Sum1 : Sum  Inputs=|+-  InputSameDT=on  SaturateOnIntegerOverflow=on  OutDataTypeStr=Inherit: Same as first input
  Switch2 : Switch  Threshold=0.5  SaturateOnIntegerOverflow=on  InputSameDT=on
  Detrended Output : Outport
  wires:
  Switch2/1 -> Detrended Output/1
  Detrending/1 -> Switch2/2, Compare To Constant/1
  Subsystem/1(Out2) -> Sum1/2
  Constant1/1 -> Switch2/1
  Input/1 -> Sum1/1, Subsystem/1(In1)
  Sum1/1 -> Switch2/3
  Compare To Constant/1 -> Subsystem/Enable

== system KF_3_gdl_AHRS_Dataset2/MPU AHRS3/debias MPU/Gyros Detrend/Detrend2 ==
  Input : Inport
  Detrending : Inport  Port=2
  Compare To Constant : simulink/Logic and Bit Operations/Compare To Constant  relop=>=  const=0.5  OutDataTypeStr=boolean
  Constant1 : Constant  Value=0  OutDataTypeStr=single
  Subsystem : Subsystem  TreatAsAtomicUnit=on
  Sum1 : Sum  Inputs=|+-  InputSameDT=on  SaturateOnIntegerOverflow=on  OutDataTypeStr=Inherit: Same as first input
  Switch2 : Switch  Threshold=0.5  SaturateOnIntegerOverflow=on  InputSameDT=on
  Detrended Output : Outport
  wires:
  Switch2/1 -> Detrended Output/1
  Detrending/1 -> Switch2/2, Compare To Constant/1
  Subsystem/1(Out2) -> Sum1/2
  Constant1/1 -> Switch2/1
  Input/1 -> Sum1/1, Subsystem/1(In1)
  Sum1/1 -> Switch2/3
  Compare To Constant/1 -> Subsystem/Enable

== system KF_3_gdl_AHRS_Dataset2/MPU AHRS3/debias MPU/Gyros Detrend/Detrend3 ==
  Input : Inport
  Detrending : Inport  Port=2
  Compare To Constant : simulink/Logic and Bit Operations/Compare To Constant  relop=>=  const=0.5  OutDataTypeStr=boolean
  Constant1 : Constant  Value=0  OutDataTypeStr=single
  Subsystem : Subsystem  TreatAsAtomicUnit=on
  Sum1 : Sum  Inputs=|+-  InputSameDT=on  SaturateOnIntegerOverflow=on  OutDataTypeStr=Inherit: Same as first input
  Switch2 : Switch  Threshold=0.5  SaturateOnIntegerOverflow=on  InputSameDT=on
  Detrended Output : Outport
  wires:
  Compare To Constant/1 -> Subsystem/Enable
  Sum1/1 -> Switch2/3
  Input/1 -> Subsystem/1(In1), Sum1/1
  Constant1/1 -> Switch2/1
  Subsystem/1(Out2) -> Sum1/2
  Detrending/1 -> Compare To Constant/1, Switch2/2
  Switch2/1 -> Detrended Output/1

== system KF_3_gdl_AHRS_Dataset2/MPU AHRS4/debias MPU/Acceleration Detrend /Detrend ==
  Input : Inport
  Detrending : Inport  Port=2
  Compare To Constant : simulink/Logic and Bit Operations/Compare To Constant  relop=>=  const=0.5  OutDataTypeStr=boolean
  Constant1 : Constant  Value=0  OutDataTypeStr=single
  Subsystem : Subsystem  TreatAsAtomicUnit=on
  Sum1 : Sum  Inputs=|+-  InputSameDT=on  SaturateOnIntegerOverflow=on  OutDataTypeStr=Inherit: Same as first input
  Switch2 : Switch  Threshold=0.5  SaturateOnIntegerOverflow=on  InputSameDT=on
  Detrended Output : Outport
  wires:
  Switch2/1 -> Detrended Output/1
  Detrending/1 -> Switch2/2, Compare To Constant/1
  Subsystem/1(Out2) -> Sum1/2
  Constant1/1 -> Switch2/1
  Input/1 -> Sum1/1, Subsystem/1(In1)
  Sum1/1 -> Switch2/3
  Compare To Constant/1 -> Subsystem/Enable

== system KF_3_gdl_AHRS_Dataset2/MPU AHRS4/debias MPU/Acceleration Detrend /Detrend1 ==
  Input : Inport
  Detrending : Inport  Port=2
  Compare To Constant : simulink/Logic and Bit Operations/Compare To Constant  relop=>=  const=0.5  OutDataTypeStr=boolean
  Constant1 : Constant  Value=0  OutDataTypeStr=single
  Subsystem : Subsystem  TreatAsAtomicUnit=on
  Sum1 : Sum  Inputs=|+-  InputSameDT=on  SaturateOnIntegerOverflow=on  OutDataTypeStr=Inherit: Same as first input
  Switch2 : Switch  Threshold=0.5  SaturateOnIntegerOverflow=on  InputSameDT=on
  Detrended Output : Outport
  wires:
  Compare To Constant/1 -> Subsystem/Enable
  Sum1/1 -> Switch2/3
  Input/1 -> Subsystem/1(In1), Sum1/1
  Constant1/1 -> Switch2/1
  Subsystem/1(Out2) -> Sum1/2
  Detrending/1 -> Compare To Constant/1, Switch2/2
  Switch2/1 -> Detrended Output/1

== system KF_3_gdl_AHRS_Dataset2/MPU AHRS4/debias MPU/Acceleration Detrend /Detrend3 ==
  Input : Inport
  Detrending : Inport  Port=2
  Compare To Constant : simulink/Logic and Bit Operations/Compare To Constant  relop=>=  const=0.5  OutDataTypeStr=boolean
  Constant1 : Constant  Value=0  OutDataTypeStr=single
  Constant2 : Constant  Value=9.81  OutDataTypeStr=single
  Subsystem : Subsystem  TreatAsAtomicUnit=on
  Sum1 : Sum  Inputs=|+--  InputSameDT=on  SaturateOnIntegerOverflow=on  OutDataTypeStr=Inherit: Same as first input
  Switch2 : Switch  Threshold=0.5  SaturateOnIntegerOverflow=on  InputSameDT=on
  Detrended Output : Outport
  wires:
  Switch2/1 -> Detrended Output/1
  Detrending/1 -> Switch2/2, Compare To Constant/1
  Subsystem/1(Out2) -> Sum1/2
  Constant1/1 -> Switch2/1
  Input/1 -> Sum1/1, Subsystem/1(In1)
  Sum1/1 -> Switch2/3
  Compare To Constant/1 -> Subsystem/Enable
  Constant2/1 -> Sum1/3

== system KF_3_gdl_AHRS_Dataset2/MPU AHRS4/debias MPU/Gyros Detrend/Detrend ==
  Input : Inport
  Detrending : Inport  Port=2
  Compare To Constant : simulink/Logic and Bit Operations/Compare To Constant  relop=>=  const=0.5  OutDataTypeStr=boolean
  Constant1 : Constant  Value=0  OutDataTypeStr=single
  Subsystem : Subsystem  TreatAsAtomicUnit=on
  Sum1 : Sum  Inputs=|+-  InputSameDT=on  SaturateOnIntegerOverflow=on  OutDataTypeStr=Inherit: Same as first input
  Switch2 : Switch  Threshold=0.5  SaturateOnIntegerOverflow=on  InputSameDT=on
  Detrended Output : Outport
  wires:
  Switch2/1 -> Detrended Output/1
  Detrending/1 -> Switch2/2, Compare To Constant/1
  Subsystem/1(Out2) -> Sum1/2
  Constant1/1 -> Switch2/1
  Input/1 -> Sum1/1, Subsystem/1(In1)
  Sum1/1 -> Switch2/3
  Compare To Constant/1 -> Subsystem/Enable

== system KF_3_gdl_AHRS_Dataset2/MPU AHRS4/debias MPU/Gyros Detrend/Detrend2 ==
  Input : Inport
  Detrending : Inport  Port=2
  Compare To Constant : simulink/Logic and Bit Operations/Compare To Constant  relop=>=  const=0.5  OutDataTypeStr=boolean
  Constant1 : Constant  Value=0  OutDataTypeStr=single
  Subsystem : Subsystem  TreatAsAtomicUnit=on
  Sum1 : Sum  Inputs=|+-  InputSameDT=on  SaturateOnIntegerOverflow=on  OutDataTypeStr=Inherit: Same as first input
  Switch2 : Switch  Threshold=0.5  SaturateOnIntegerOverflow=on  InputSameDT=on
  Detrended Output : Outport
  wires:
  Switch2/1 -> Detrended Output/1
  Detrending/1 -> Switch2/2, Compare To Constant/1
  Subsystem/1(Out2) -> Sum1/2
  Constant1/1 -> Switch2/1
  Input/1 -> Sum1/1, Subsystem/1(In1)
  Sum1/1 -> Switch2/3
  Compare To Constant/1 -> Subsystem/Enable

== system KF_3_gdl_AHRS_Dataset2/MPU AHRS4/debias MPU/Gyros Detrend/Detrend3 ==
  Input : Inport
  Detrending : Inport  Port=2
  Compare To Constant : simulink/Logic and Bit Operations/Compare To Constant  relop=>=  const=0.5  OutDataTypeStr=boolean
  Constant1 : Constant  Value=0  OutDataTypeStr=single
  Subsystem : Subsystem  TreatAsAtomicUnit=on
  Sum1 : Sum  Inputs=|+-  InputSameDT=on  SaturateOnIntegerOverflow=on  OutDataTypeStr=Inherit: Same as first input
  Switch2 : Switch  Threshold=0.5  SaturateOnIntegerOverflow=on  InputSameDT=on
  Detrended Output : Outport
  wires:
  Compare To Constant/1 -> Subsystem/Enable
  Sum1/1 -> Switch2/3
  Input/1 -> Subsystem/1(In1), Sum1/1
  Constant1/1 -> Switch2/1
  Subsystem/1(Out2) -> Sum1/2
  Detrending/1 -> Compare To Constant/1, Switch2/2
  Switch2/1 -> Detrended Output/1

== system KF_3_gdl_AHRS_Dataset2/MPU AHRS1/debias MPU/Acceleration Detrend /Detrend/Subsystem ==
  In1 : Inport
  Enable : EnablePort
  Constant : Constant  OutDataTypeStr=single
  Discrete-Time Integrator : DiscreteIntegrator  SampleTime=ST  ICPrevOutput=DiscIntNeverNeededParam  ICPrevScaledInput=DiscIntNeverNeededParam
  Discrete-Time Integrator1 : DiscreteIntegrator  InitialCondition=eps  SampleTime=ST  ICPrevOutput=DiscIntNeverNeededParam  ICPrevScaledInput=DiscIntNeverNeededParam
  Product1 : Product  Inputs=*/  InputSameDT=on  RndMeth=Zero  SaturateOnIntegerOverflow=on  OutDataTypeStr=Inherit: Same as first input
  Out2 : Outport
  wires:
  Constant/1 -> Discrete-Time Integrator1/1
  Discrete-Time Integrator1/1 -> Product1/2
  Product1/1 -> Out2/1
  Discrete-Time Integrator/1 -> Product1/1
  In1/1 -> Discrete-Time Integrator/1

== system KF_3_gdl_AHRS_Dataset2/MPU AHRS1/debias MPU/Acceleration Detrend /Detrend1/Subsystem ==
  In1 : Inport
  Enable : EnablePort
  Constant : Constant  OutDataTypeStr=single
  Discrete-Time Integrator : DiscreteIntegrator  SampleTime=ST  ICPrevOutput=DiscIntNeverNeededParam  ICPrevScaledInput=DiscIntNeverNeededParam
  Discrete-Time Integrator1 : DiscreteIntegrator  InitialCondition=eps  SampleTime=ST  ICPrevOutput=DiscIntNeverNeededParam  ICPrevScaledInput=DiscIntNeverNeededParam
  Product1 : Product  Inputs=*/  InputSameDT=on  RndMeth=Zero  SaturateOnIntegerOverflow=on  OutDataTypeStr=Inherit: Same as first input
  Out2 : Outport
  wires:
  In1/1 -> Discrete-Time Integrator/1
  Discrete-Time Integrator/1 -> Product1/1
  Product1/1 -> Out2/1
  Discrete-Time Integrator1/1 -> Product1/2
  Constant/1 -> Discrete-Time Integrator1/1

== system KF_3_gdl_AHRS_Dataset2/MPU AHRS1/debias MPU/Acceleration Detrend /Detrend3/Subsystem ==
  In1 : Inport
  Enable : EnablePort
  Constant : Constant  OutDataTypeStr=single
  Discrete-Time Integrator : DiscreteIntegrator  SampleTime=ST  ICPrevOutput=DiscIntNeverNeededParam  ICPrevScaledInput=DiscIntNeverNeededParam
  Discrete-Time Integrator1 : DiscreteIntegrator  InitialCondition=eps  SampleTime=ST  ICPrevOutput=DiscIntNeverNeededParam  ICPrevScaledInput=DiscIntNeverNeededParam
  Product1 : Product  Inputs=*/  InputSameDT=on  RndMeth=Zero  SaturateOnIntegerOverflow=on  OutDataTypeStr=Inherit: Same as first input
  Out2 : Outport
  wires:
  Constant/1 -> Discrete-Time Integrator1/1
  Discrete-Time Integrator1/1 -> Product1/2
  Product1/1 -> Out2/1
  Discrete-Time Integrator/1 -> Product1/1
  In1/1 -> Discrete-Time Integrator/1

== system KF_3_gdl_AHRS_Dataset2/MPU AHRS1/debias MPU/Gyros Detrend/Detrend/Subsystem ==
  In1 : Inport
  Enable : EnablePort
  Constant : Constant  OutDataTypeStr=single
  Discrete-Time Integrator : DiscreteIntegrator  SampleTime=ST  ICPrevOutput=DiscIntNeverNeededParam  ICPrevScaledInput=DiscIntNeverNeededParam
  Discrete-Time Integrator1 : DiscreteIntegrator  InitialCondition=eps  SampleTime=ST  ICPrevOutput=DiscIntNeverNeededParam  ICPrevScaledInput=DiscIntNeverNeededParam
  Product1 : Product  Inputs=*/  InputSameDT=on  RndMeth=Zero  SaturateOnIntegerOverflow=on  OutDataTypeStr=Inherit: Same as first input
  Out2 : Outport
  wires:
  Constant/1 -> Discrete-Time Integrator1/1
  Discrete-Time Integrator1/1 -> Product1/2
  Product1/1 -> Out2/1
  Discrete-Time Integrator/1 -> Product1/1
  In1/1 -> Discrete-Time Integrator/1

== system KF_3_gdl_AHRS_Dataset2/MPU AHRS1/debias MPU/Gyros Detrend/Detrend2/Subsystem ==
  In1 : Inport
  Enable : EnablePort
  Constant : Constant  OutDataTypeStr=single
  Discrete-Time Integrator : DiscreteIntegrator  SampleTime=ST  ICPrevOutput=DiscIntNeverNeededParam  ICPrevScaledInput=DiscIntNeverNeededParam
  Discrete-Time Integrator1 : DiscreteIntegrator  InitialCondition=eps  SampleTime=ST  ICPrevOutput=DiscIntNeverNeededParam  ICPrevScaledInput=DiscIntNeverNeededParam
  Product1 : Product  Inputs=*/  InputSameDT=on  RndMeth=Zero  SaturateOnIntegerOverflow=on  OutDataTypeStr=Inherit: Same as first input
  Out2 : Outport
  wires:
  Constant/1 -> Discrete-Time Integrator1/1
  Discrete-Time Integrator1/1 -> Product1/2
  Product1/1 -> Out2/1
  Discrete-Time Integrator/1 -> Product1/1
  In1/1 -> Discrete-Time Integrator/1

== system KF_3_gdl_AHRS_Dataset2/MPU AHRS1/debias MPU/Gyros Detrend/Detrend3/Subsystem ==
  In1 : Inport
  Enable : EnablePort
  Constant : Constant  OutDataTypeStr=single
  Discrete-Time Integrator : DiscreteIntegrator  SampleTime=ST  ICPrevOutput=DiscIntNeverNeededParam  ICPrevScaledInput=DiscIntNeverNeededParam
  Discrete-Time Integrator1 : DiscreteIntegrator  InitialCondition=eps  SampleTime=ST  ICPrevOutput=DiscIntNeverNeededParam  ICPrevScaledInput=DiscIntNeverNeededParam
  Product1 : Product  Inputs=*/  InputSameDT=on  RndMeth=Zero  SaturateOnIntegerOverflow=on  OutDataTypeStr=Inherit: Same as first input
  Out2 : Outport
  wires:
  In1/1 -> Discrete-Time Integrator/1
  Discrete-Time Integrator/1 -> Product1/1
  Product1/1 -> Out2/1
  Discrete-Time Integrator1/1 -> Product1/2
  Constant/1 -> Discrete-Time Integrator1/1

== system KF_3_gdl_AHRS_Dataset2/MPU AHRS3/debias MPU/Acceleration Detrend /Detrend/Subsystem ==
  In1 : Inport
  Enable : EnablePort
  Constant : Constant  OutDataTypeStr=single
  Discrete-Time Integrator : DiscreteIntegrator  SampleTime=ST  ICPrevOutput=DiscIntNeverNeededParam  ICPrevScaledInput=DiscIntNeverNeededParam
  Discrete-Time Integrator1 : DiscreteIntegrator  InitialCondition=eps  SampleTime=ST  ICPrevOutput=DiscIntNeverNeededParam  ICPrevScaledInput=DiscIntNeverNeededParam
  Product1 : Product  Inputs=*/  InputSameDT=on  RndMeth=Zero  SaturateOnIntegerOverflow=on  OutDataTypeStr=Inherit: Same as first input
  Out2 : Outport
  wires:
  Constant/1 -> Discrete-Time Integrator1/1
  Discrete-Time Integrator1/1 -> Product1/2
  Product1/1 -> Out2/1
  Discrete-Time Integrator/1 -> Product1/1
  In1/1 -> Discrete-Time Integrator/1

== system KF_3_gdl_AHRS_Dataset2/MPU AHRS3/debias MPU/Acceleration Detrend /Detrend1/Subsystem ==
  In1 : Inport
  Enable : EnablePort
  Constant : Constant  OutDataTypeStr=single
  Discrete-Time Integrator : DiscreteIntegrator  SampleTime=ST  ICPrevOutput=DiscIntNeverNeededParam  ICPrevScaledInput=DiscIntNeverNeededParam
  Discrete-Time Integrator1 : DiscreteIntegrator  InitialCondition=eps  SampleTime=ST  ICPrevOutput=DiscIntNeverNeededParam  ICPrevScaledInput=DiscIntNeverNeededParam
  Product1 : Product  Inputs=*/  InputSameDT=on  RndMeth=Zero  SaturateOnIntegerOverflow=on  OutDataTypeStr=Inherit: Same as first input
  Out2 : Outport
  wires:
  In1/1 -> Discrete-Time Integrator/1
  Discrete-Time Integrator/1 -> Product1/1
  Product1/1 -> Out2/1
  Discrete-Time Integrator1/1 -> Product1/2
  Constant/1 -> Discrete-Time Integrator1/1

== system KF_3_gdl_AHRS_Dataset2/MPU AHRS3/debias MPU/Acceleration Detrend /Detrend3/Subsystem ==
  In1 : Inport
  Enable : EnablePort
  Constant : Constant  OutDataTypeStr=single
  Discrete-Time Integrator : DiscreteIntegrator  SampleTime=ST  ICPrevOutput=DiscIntNeverNeededParam  ICPrevScaledInput=DiscIntNeverNeededParam
  Discrete-Time Integrator1 : DiscreteIntegrator  InitialCondition=eps  SampleTime=ST  ICPrevOutput=DiscIntNeverNeededParam  ICPrevScaledInput=DiscIntNeverNeededParam
  Product1 : Product  Inputs=*/  InputSameDT=on  RndMeth=Zero  SaturateOnIntegerOverflow=on  OutDataTypeStr=Inherit: Same as first input
  Out2 : Outport
  wires:
  Constant/1 -> Discrete-Time Integrator1/1
  Discrete-Time Integrator1/1 -> Product1/2
  Product1/1 -> Out2/1
  Discrete-Time Integrator/1 -> Product1/1
  In1/1 -> Discrete-Time Integrator/1

== system KF_3_gdl_AHRS_Dataset2/MPU AHRS3/debias MPU/Gyros Detrend/Detrend/Subsystem ==
  In1 : Inport
  Enable : EnablePort
  Constant : Constant  OutDataTypeStr=single
  Discrete-Time Integrator : DiscreteIntegrator  SampleTime=ST  ICPrevOutput=DiscIntNeverNeededParam  ICPrevScaledInput=DiscIntNeverNeededParam
  Discrete-Time Integrator1 : DiscreteIntegrator  InitialCondition=eps  SampleTime=ST  ICPrevOutput=DiscIntNeverNeededParam  ICPrevScaledInput=DiscIntNeverNeededParam
  Product1 : Product  Inputs=*/  InputSameDT=on  RndMeth=Zero  SaturateOnIntegerOverflow=on  OutDataTypeStr=Inherit: Same as first input
  Out2 : Outport
  wires:
  Constant/1 -> Discrete-Time Integrator1/1
  Discrete-Time Integrator1/1 -> Product1/2
  Product1/1 -> Out2/1
  Discrete-Time Integrator/1 -> Product1/1
  In1/1 -> Discrete-Time Integrator/1

== system KF_3_gdl_AHRS_Dataset2/MPU AHRS3/debias MPU/Gyros Detrend/Detrend2/Subsystem ==
  In1 : Inport
  Enable : EnablePort
  Constant : Constant  OutDataTypeStr=single
  Discrete-Time Integrator : DiscreteIntegrator  SampleTime=ST  ICPrevOutput=DiscIntNeverNeededParam  ICPrevScaledInput=DiscIntNeverNeededParam
  Discrete-Time Integrator1 : DiscreteIntegrator  InitialCondition=eps  SampleTime=ST  ICPrevOutput=DiscIntNeverNeededParam  ICPrevScaledInput=DiscIntNeverNeededParam
  Product1 : Product  Inputs=*/  InputSameDT=on  RndMeth=Zero  SaturateOnIntegerOverflow=on  OutDataTypeStr=Inherit: Same as first input
  Out2 : Outport
  wires:
  Constant/1 -> Discrete-Time Integrator1/1
  Discrete-Time Integrator1/1 -> Product1/2
  Product1/1 -> Out2/1
  Discrete-Time Integrator/1 -> Product1/1
  In1/1 -> Discrete-Time Integrator/1

== system KF_3_gdl_AHRS_Dataset2/MPU AHRS3/debias MPU/Gyros Detrend/Detrend3/Subsystem ==
  In1 : Inport
  Enable : EnablePort
  Constant : Constant  OutDataTypeStr=single
  Discrete-Time Integrator : DiscreteIntegrator  SampleTime=ST  ICPrevOutput=DiscIntNeverNeededParam  ICPrevScaledInput=DiscIntNeverNeededParam
  Discrete-Time Integrator1 : DiscreteIntegrator  InitialCondition=eps  SampleTime=ST  ICPrevOutput=DiscIntNeverNeededParam  ICPrevScaledInput=DiscIntNeverNeededParam
  Product1 : Product  Inputs=*/  InputSameDT=on  RndMeth=Zero  SaturateOnIntegerOverflow=on  OutDataTypeStr=Inherit: Same as first input
  Out2 : Outport
  wires:
  In1/1 -> Discrete-Time Integrator/1
  Discrete-Time Integrator/1 -> Product1/1
  Product1/1 -> Out2/1
  Discrete-Time Integrator1/1 -> Product1/2
  Constant/1 -> Discrete-Time Integrator1/1

== system KF_3_gdl_AHRS_Dataset2/MPU AHRS4/debias MPU/Acceleration Detrend /Detrend/Subsystem ==
  In1 : Inport
  Enable : EnablePort
  Constant : Constant  OutDataTypeStr=single
  Discrete-Time Integrator : DiscreteIntegrator  SampleTime=ST  ICPrevOutput=DiscIntNeverNeededParam  ICPrevScaledInput=DiscIntNeverNeededParam
  Discrete-Time Integrator1 : DiscreteIntegrator  InitialCondition=eps  SampleTime=ST  ICPrevOutput=DiscIntNeverNeededParam  ICPrevScaledInput=DiscIntNeverNeededParam
  Product1 : Product  Inputs=*/  InputSameDT=on  RndMeth=Zero  SaturateOnIntegerOverflow=on  OutDataTypeStr=Inherit: Same as first input
  Out2 : Outport
  wires:
  Constant/1 -> Discrete-Time Integrator1/1
  Discrete-Time Integrator1/1 -> Product1/2
  Product1/1 -> Out2/1
  Discrete-Time Integrator/1 -> Product1/1
  In1/1 -> Discrete-Time Integrator/1

== system KF_3_gdl_AHRS_Dataset2/MPU AHRS4/debias MPU/Acceleration Detrend /Detrend1/Subsystem ==
  In1 : Inport
  Enable : EnablePort
  Constant : Constant  OutDataTypeStr=single
  Discrete-Time Integrator : DiscreteIntegrator  SampleTime=ST  ICPrevOutput=DiscIntNeverNeededParam  ICPrevScaledInput=DiscIntNeverNeededParam
  Discrete-Time Integrator1 : DiscreteIntegrator  InitialCondition=eps  SampleTime=ST  ICPrevOutput=DiscIntNeverNeededParam  ICPrevScaledInput=DiscIntNeverNeededParam
  Product1 : Product  Inputs=*/  InputSameDT=on  RndMeth=Zero  SaturateOnIntegerOverflow=on  OutDataTypeStr=Inherit: Same as first input
  Out2 : Outport
  wires:
  In1/1 -> Discrete-Time Integrator/1
  Discrete-Time Integrator/1 -> Product1/1
  Product1/1 -> Out2/1
  Discrete-Time Integrator1/1 -> Product1/2
  Constant/1 -> Discrete-Time Integrator1/1

== system KF_3_gdl_AHRS_Dataset2/MPU AHRS4/debias MPU/Acceleration Detrend /Detrend3/Subsystem ==
  In1 : Inport
  Enable : EnablePort
  Constant : Constant  OutDataTypeStr=single
  Discrete-Time Integrator : DiscreteIntegrator  SampleTime=ST  ICPrevOutput=DiscIntNeverNeededParam  ICPrevScaledInput=DiscIntNeverNeededParam
  Discrete-Time Integrator1 : DiscreteIntegrator  InitialCondition=eps  SampleTime=ST  ICPrevOutput=DiscIntNeverNeededParam  ICPrevScaledInput=DiscIntNeverNeededParam
  Product1 : Product  Inputs=*/  InputSameDT=on  RndMeth=Zero  SaturateOnIntegerOverflow=on  OutDataTypeStr=Inherit: Same as first input
  Out2 : Outport
  wires:
  Constant/1 -> Discrete-Time Integrator1/1
  Discrete-Time Integrator1/1 -> Product1/2
  Product1/1 -> Out2/1
  Discrete-Time Integrator/1 -> Product1/1
  In1/1 -> Discrete-Time Integrator/1

== system KF_3_gdl_AHRS_Dataset2/MPU AHRS4/debias MPU/Gyros Detrend/Detrend/Subsystem ==
  In1 : Inport
  Enable : EnablePort
  Constant : Constant  OutDataTypeStr=single
  Discrete-Time Integrator : DiscreteIntegrator  SampleTime=ST  ICPrevOutput=DiscIntNeverNeededParam  ICPrevScaledInput=DiscIntNeverNeededParam
  Discrete-Time Integrator1 : DiscreteIntegrator  InitialCondition=eps  SampleTime=ST  ICPrevOutput=DiscIntNeverNeededParam  ICPrevScaledInput=DiscIntNeverNeededParam
  Product1 : Product  Inputs=*/  InputSameDT=on  RndMeth=Zero  SaturateOnIntegerOverflow=on  OutDataTypeStr=Inherit: Same as first input
  Out2 : Outport
  wires:
  Constant/1 -> Discrete-Time Integrator1/1
  Discrete-Time Integrator1/1 -> Product1/2
  Product1/1 -> Out2/1
  Discrete-Time Integrator/1 -> Product1/1
  In1/1 -> Discrete-Time Integrator/1

== system KF_3_gdl_AHRS_Dataset2/MPU AHRS4/debias MPU/Gyros Detrend/Detrend2/Subsystem ==
  In1 : Inport
  Enable : EnablePort
  Constant : Constant  OutDataTypeStr=single
  Discrete-Time Integrator : DiscreteIntegrator  SampleTime=ST  ICPrevOutput=DiscIntNeverNeededParam  ICPrevScaledInput=DiscIntNeverNeededParam
  Discrete-Time Integrator1 : DiscreteIntegrator  InitialCondition=eps  SampleTime=ST  ICPrevOutput=DiscIntNeverNeededParam  ICPrevScaledInput=DiscIntNeverNeededParam
  Product1 : Product  Inputs=*/  InputSameDT=on  RndMeth=Zero  SaturateOnIntegerOverflow=on  OutDataTypeStr=Inherit: Same as first input
  Out2 : Outport
  wires:
  Constant/1 -> Discrete-Time Integrator1/1
  Discrete-Time Integrator1/1 -> Product1/2
  Product1/1 -> Out2/1
  Discrete-Time Integrator/1 -> Product1/1
  In1/1 -> Discrete-Time Integrator/1

== system KF_3_gdl_AHRS_Dataset2/MPU AHRS4/debias MPU/Gyros Detrend/Detrend3/Subsystem ==
  In1 : Inport
  Enable : EnablePort
  Constant : Constant  OutDataTypeStr=single
  Discrete-Time Integrator : DiscreteIntegrator  SampleTime=ST  ICPrevOutput=DiscIntNeverNeededParam  ICPrevScaledInput=DiscIntNeverNeededParam
  Discrete-Time Integrator1 : DiscreteIntegrator  InitialCondition=eps  SampleTime=ST  ICPrevOutput=DiscIntNeverNeededParam  ICPrevScaledInput=DiscIntNeverNeededParam
  Product1 : Product  Inputs=*/  InputSameDT=on  RndMeth=Zero  SaturateOnIntegerOverflow=on  OutDataTypeStr=Inherit: Same as first input
  Out2 : Outport
  wires:
  In1/1 -> Discrete-Time Integrator/1
  Discrete-Time Integrator/1 -> Product1/1
  Product1/1 -> Out2/1
  Discrete-Time Integrator1/1 -> Product1/2
  Constant/1 -> Discrete-Time Integrator1/1
